simulink model "untitled"  (R2018a)
settings: Solver=ode45  StartTime=0.0  StopTime=1  RelTol=1e-3
libraries: powerlib x4, simulink x2, electricdrivelib x1, spsDrivesSpeedControllerModel x1
settings Model: Creator=HP  LastModifiedBy=HP

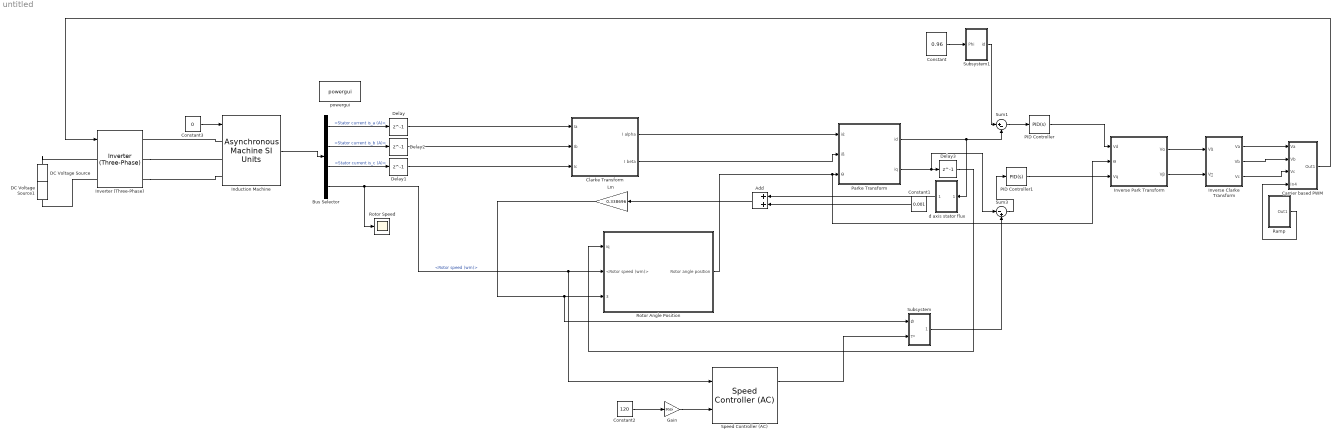
== system untitled ==
  Add : Sum
  Bus Selector : BusSelector  OutputSignals=Stator measurements.Stator current is_a (A),Stator measurements.Stator current is_b (A),Stator measurements.Stator current is_c (A),Mechanical.Rotor speed (wm)
  Carrier based PWM : Subsystem
  Clarke Transform : Subsystem
  Constant : Constant  Value=0.96
  Constant1 : Constant  Value=0.001
  Constant2 : Constant  Value=120
  Constant3 : Constant  Value=0
  DC Voltage Source : powerlib/Electrical Sources/DC Voltage Source  Amplitude=250  Measurements=None
  DC Voltage Source1 : powerlib/Electrical Sources/DC Voltage Source  Amplitude=250  Measurements=None
  Delay{,1..3} (4 alike) : Delay  DelayLength=1  InitialCondition=0
  Gain : Gain  Gain=30/pi
  "Induction Machine " : powerlib/Machines/Asynchronous Machine SI Units  RotorType=Squirrel-cage  PresetModel=No  MechanicalLoad=Torque Tm  ShowDetailedParameters=on  ReferenceFrame=Rotor  Units=SI  MeasurementBus=off  NominalParameters=[1.845e+04 460 50]  Stator=[0.6837 0.004152]  Rotor=[0.451 0.004152]  Cage1=[0.4155 0.002066]  Cage2=[0.4168 0.0003495]  Lm=0.1486  Mechanical=[0.05 0.005879 2]  PolePairs=2  InitialConditions=[1 0 0 0 0 0 0 0]  SimulateSaturation=off  Saturation=[14.03593122, 27.81365428, 53.79336849, 72.68890987, 97.98006896, 148.6815601, 215.7428561, 302.9841135, 428.7778367 ; 230, 322, 414, 460, 506, 552, 598, 644, 690]  LoadFlowParameters=1492000  TsPowergui=0  TsBlock=-1  IterativeModel=Trapezoidal non iterative  IterativeDiscreteModel=Trapezoidal non iterative  Pmec=1.492e+006
  Inverse Clarke Transform : Subsystem
  Inverse Park Transform : Subsystem
  Inverter (Three-Phase) : electricdrivelib/Fundamental Drive Blocks/Inverter (Three-Phase)  OverrideUsingVariant=Detailed  detailLevel=Detailed  driveType=Field-oriented control  Ts=2e-6  SnubberResistance=10e3  SnubberCapacitance=inf  Device=IGBT / Diodes  Ron=1e-3  ForwardVoltages=[1.2,1.2]  GTOparameters=[1e-6,2e-6]  IGBTparameters=[1e-6,2e-6]  Measurements=All voltages and currents  converterType=Inverter  SourceFrequency=60  ReferenceFrame=Rotor  dqInductances=[8.5e-3,8.5e-3]  Inductance=8.5e-3  Ls=0  Resistance=0.2  Flux=0.175  Stator_sm=[2.01e-3,4.289e-4,4.477e-3,1.354e-3]  Stator_im=[14.85e-3,0.3027e-3]  Rotor=[9.295e-3,0.3027e-3]  Lm=10.46e-3  p=4
      settings: AttributesFormatString=%<BlockChoice>  SourceProductName=Simscape Power Systems  SourceProductBaseCode=PS
  Lm : Gain  Gain=0.338696
  PID Controller : simulink/Continuous/PID Controller  Controller=PID  TimeDomain=Continuous-time  SampleTime=-1  IntegratorMethod=Forward Euler  FilterMethod=Forward Euler  Form=Parallel  UseFilter=on  ControllerParametersSource=internal  P=5000  I=200  D=0  N=100  InitialConditionSource=internal  InitialConditionForIntegrator=0  InitialConditionForFilter=0  ExternalReset=none  LimitOutput=off  UpperSaturationLimit=inf  LowerSaturationLimit=-inf  LinearizeAsGain=on  AntiWindupMode=none  Kb=1  TrackingMode=off  Kt=1  PParamMin=[]  PParamMax=[]  IParamMin=[]  IParamMax=[]  DParamMin=[]  DParamMax=[]  NParamMin=[]  NParamMax=[]  KbParamMin=[]  KbParamMax=[]  KtParamMin=[]  KtParamMax=[]  POutMin=[]  POutMax=[]  IOutMin=[]  IOutMax=[]  DOutMin=[]  DOutMax=[]  NOutMin=[]  NOutMax=[]  KbOutMin=[]  KbOutMax=[]  KtOutMin=[]  KtOutMax=[]  IntegratorOutMin=[]  IntegratorOutMax=[]  FilterOutMin=[]  FilterOutMax=[]  SumOutMin=[]  SumOutMax=[]  SumI1OutMin=[]  SumI1OutMax=[]  SumI2OutMin=[]  SumI2OutMax=[]  SumI3OutMin=[]  SumI3OutMax=[]  SumDOutMin=[]  SumDOutMax=[]  SaturationOutMin=[]  SaturationOutMax=[]  IntegratorContinuousStateAttributes=''  IntegratorStateMustResolveToSignalObject=off  IntegratorRTWStateStorageClass=Auto  FilterContinuousStateAttributes=''  FilterStateMustResolveToSignalObject=off  FilterRTWStateStorageClass=Auto  DifferentiatorICPrevScaledInput=0  DifferentiatorOutMin=[]  DifferentiatorOutMax=[]  FilterDiffOutCoefMin=[]  FilterDiffOutCoefMax=[]  SumDenOutMin=[]  SumDenOutMax=[]  SumNumOutMin=[]  SumNumOutMax=[]  ReciprocalOutMin=[]  ReciprocalOutMax=[]  DivideOutMin=[]  DivideOutMax=[]  TunerSelectOption=Transfer Function Based (PID Tuner App)
  PID Controller1 : simulink/Continuous/PID Controller  Controller=PID  TimeDomain=Continuous-time  SampleTime=-1  IntegratorMethod=Forward Euler  FilterMethod=Forward Euler  Form=Parallel  UseFilter=on  ControllerParametersSource=internal  P=5000  I=200  D=0  N=100  InitialConditionSource=internal  InitialConditionForIntegrator=0  InitialConditionForFilter=0  ExternalReset=none  LimitOutput=off  UpperSaturationLimit=inf  LowerSaturationLimit=-inf  LinearizeAsGain=on  AntiWindupMode=none  Kb=1  TrackingMode=off  Kt=1  PParamMin=[]  PParamMax=[]  IParamMin=[]  IParamMax=[]  DParamMin=[]  DParamMax=[]  NParamMin=[]  NParamMax=[]  KbParamMin=[]  KbParamMax=[]  KtParamMin=[]  KtParamMax=[]  POutMin=[]  POutMax=[]  IOutMin=[]  IOutMax=[]  DOutMin=[]  DOutMax=[]  NOutMin=[]  NOutMax=[]  KbOutMin=[]  KbOutMax=[]  KtOutMin=[]  KtOutMax=[]  IntegratorOutMin=[]  IntegratorOutMax=[]  FilterOutMin=[]  FilterOutMax=[]  SumOutMin=[]  SumOutMax=[]  SumI1OutMin=[]  SumI1OutMax=[]  SumI2OutMin=[]  SumI2OutMax=[]  SumI3OutMin=[]  SumI3OutMax=[]  SumDOutMin=[]  SumDOutMax=[]  SaturationOutMin=[]  SaturationOutMax=[]  IntegratorContinuousStateAttributes=''  IntegratorStateMustResolveToSignalObject=off  IntegratorRTWStateStorageClass=Auto  FilterContinuousStateAttributes=''  FilterStateMustResolveToSignalObject=off  FilterRTWStateStorageClass=Auto  DifferentiatorICPrevScaledInput=0  DifferentiatorOutMin=[]  DifferentiatorOutMax=[]  FilterDiffOutCoefMin=[]  FilterDiffOutCoefMax=[]  SumDenOutMin=[]  SumDenOutMax=[]  SumNumOutMin=[]  SumNumOutMax=[]  ReciprocalOutMin=[]  ReciprocalOutMax=[]  DivideOutMin=[]  DivideOutMax=[]  TunerSelectOption=Transfer Function Based (PID Tuner App)
  Parke Transform : Subsystem
  Ramp : Subsystem
  Rotor Angle Position : Subsystem
  "Rotor Speed " : Scope
  Speed Controller (AC) : spsDrivesSpeedControllerModel/Speed Controller (AC)  OverrideUsingVariant=AC345  ctrlType=Without flux reference output  SwK=Speed regulation  Ts=2e-6  ramp=[-18000000000000,18000000000000]  kp=166.2  ki=27700  fc=100  ctrl_sat=[-100,100]  Tsc=100e-6  fn=60  p=2  nf=0.3
      settings: SourceProductName=The database C:\Users\ak23510\AppData\Roaming\MathWorks\MATLAB\R2017a\slblocks_master.db is locked, or a table in the database is locked. (database is locked)
  Subsystem : Subsystem
  Subsystem1 : Subsystem
  Sum1 : Sum  Inputs=|+-
  Sum3 : Sum  Inputs=|-+
  d axis stator flux : Subsystem
  powergui : powerlib/powergui  Priority=1  SimulationMode=Discrete  SampleTime=2e-6  frequency=60  Iterations=50  frequencyindice=50  Pbase=100e6  ErrMax=1e-4  UnitsV=kV  UnitsW=MW  buscounter=0  FunctionMessages=off  echomessages=off  EnableUseOfTLC=off  CurrentSourceSwitches=off  DisableSnubberDevices=off  DisableRonSwitches=off  DisableVfSwitches=off  DisplayEquations=off  SolverType=Tustin/Backward Euler (TBE)  Interpol=off  ExternalGateDelay=off  methode=off  Ts=100  x0status=blocks  SPID=on  SwTol=0  HookPort=off  RestoreLinks=warning  ResistiveCurrentMeasurement=off  Frange=[0:2:500]  Ylog=off  Xlog=on  ShowGrid=off  save=off  variable=ZData  structure=0  ZoomFFT=off  StartTime=0.0  cycles=1  DisplayStyle=1  fundamental=60  FreqAxis=off  MaxFrequency=1000  frequencyindicesteady=1  RmsSteady=1  display=off
  wires:
  "Induction Machine "/1 -> Bus Selector/1
  Bus Selector/1 -> Delay/1  "<Stator current is_a (A)>"
  Bus Selector/2 -> Delay2/1  "<Stator current is_b (A)>"
  Bus Selector/3 -> Delay1/1  "<Stator current is_c (A)>"
  Delay/1 -> Clarke Transform/1(Ia)
  Delay2/1 -> Clarke Transform/2(Ib)
  Delay1/1 -> Clarke Transform/3(Ic)
  Clarke Transform/1(I alpha) -> Parke Transform/1("iά ")
  Clarke Transform/2(I beta) -> Parke Transform/2(iß)
  Parke Transform/1(id) -> d axis stator flux/1(In1), Sum1/2
  d axis stator flux/1(øds) -> Add/1
  Constant1/1 -> Add/2
  Add/1 -> Lm/1
  Bus Selector/4 -> "Rotor Speed "/1, Speed Controller (AC)/1, Rotor Angle Position/2(<Rotor speed (wm)>)  "<Rotor speed (wm)>"
  Lm/1 -> Subsystem/1(Ǿ), Rotor Angle Position/3(" ")
  Rotor Angle Position/1("Rotor angle position ") -> Inverse Park Transform/2(Ɵ), Parke Transform/3(Ɵ)
  Subsystem1/1("id ") -> Sum1/1
  Sum1/1 -> PID Controller/1
  Sum3/1 -> PID Controller1/1
  Subsystem/1(iq ref) -> Sum3/2
  PID Controller/1 -> Inverse Park Transform/1(Vd)
  PID Controller1/1 -> Inverse Park Transform/3(Vq)
  Inverse Park Transform/2(Vβ) -> Inverse Clarke Transform/2(Vꞵ)
  Ramp/1(Out1) -> Carrier based PWM/4(In4)
  Inverse Park Transform/1(Vα) -> Inverse Clarke Transform/1(Vἀ)
  Inverse Clarke Transform/2(Vb) -> Carrier based PWM/2(Vb)
  Inverse Clarke Transform/1(Va) -> Carrier based PWM/1(Va)
  Inverse Clarke Transform/3(Vc) -> Carrier based PWM/3(Vc)
  Carrier based PWM/1(Out1) -> Inverter (Three-Phase)/1
  Constant/1 -> Subsystem1/1(Phi)
  Gain/1 -> Speed Controller (AC)/2
  Constant2/1 -> Gain/1
  Speed Controller (AC)/1 -> Subsystem/2(T*)
  Constant3/1 -> "Induction Machine "/1
  Parke Transform/2(iq) -> Sum3/1, Delay3/1
  Delay3/1 -> Rotor Angle Position/1(iq)
  connections:
  "Induction Machine "/LConn1 -- Inverter (Three-Phase)/RConn1
  Inverter (Three-Phase)/RConn2 -- "Induction Machine "/LConn2
  Inverter (Three-Phase)/RConn3 -- "Induction Machine "/LConn3
  DC Voltage Source1/RConn1 -- DC Voltage Source/LConn1
  DC Voltage Source/RConn1 -- Inverter (Three-Phase)/LConn1
  DC Voltage Source1/LConn1 -- Inverter (Three-Phase)/LConn2

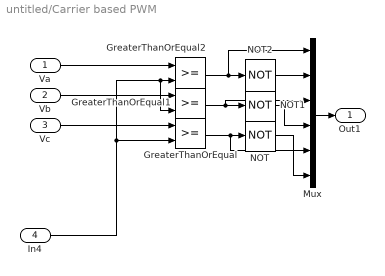
== system untitled/Carrier based PWM ==
  Va : Inport
  Vb : Inport  Port=2
  Vc : Inport  Port=3
  In4 : Inport  Port=4
  GreaterThanOrEqual : RelationalOperator  OutDataTypeStr=boolean  RndMeth=Simplest
  GreaterThanOrEqual1 : RelationalOperator  OutDataTypeStr=boolean  RndMeth=Simplest
  GreaterThanOrEqual2 : RelationalOperator  OutDataTypeStr=boolean  RndMeth=Simplest
  Mux : Mux  Inputs=6
  NOT : Logic  Operator=NOT  IconShape=distinctive  AllPortsSameDT=off  OutDataTypeStr=boolean
  NOT1 : Logic  Operator=NOT  IconShape=distinctive  AllPortsSameDT=off  OutDataTypeStr=boolean
  NOT2 : Logic  Operator=NOT  IconShape=distinctive  AllPortsSameDT=off  OutDataTypeStr=boolean
  Out1 : Outport
  wires:
  GreaterThanOrEqual1/1 -> Mux/3, NOT1/1
  GreaterThanOrEqual2/1 -> Mux/1, NOT2/1
  NOT2/1 -> Mux/2
  NOT1/1 -> Mux/4
  In4/1 -> GreaterThanOrEqual/2, GreaterThanOrEqual1/2, GreaterThanOrEqual2/2
  Va/1 -> GreaterThanOrEqual2/1
  NOT/1 -> Mux/6
  GreaterThanOrEqual/1 -> Mux/5, NOT/1
  Vb/1 -> GreaterThanOrEqual1/1
  Mux/1 -> Out1/1
  Vc/1 -> GreaterThanOrEqual/1

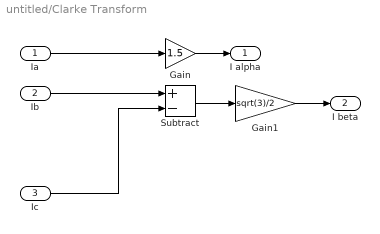
== system untitled/Clarke Transform ==
  Ia : Inport
  Ib : Inport  Port=2
  Ic : Inport  Port=3
  Gain : Gain  Gain=1.5
  Gain1 : Gain  Gain=sqrt(3)/2
  Subtract : Sum  Inputs=+-
  I alpha : Outport
  I beta : Outport  Port=2
  wires:
  Subtract/1 -> Gain1/1
  Ic/1 -> Subtract/2
  Gain1/1 -> I beta/1
  Ia/1 -> Gain/1
  Ib/1 -> Subtract/1
  Gain/1 -> I alpha/1

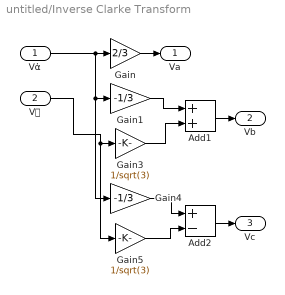
== system untitled/Inverse Clarke Transform ==
  Vἀ : Inport
  Vꞵ : Inport  Port=2
  Add1 : Sum
  Add2 : Sum  Inputs=+-
  Gain : Gain  Gain=2/3
  Gain1 : Gain  Gain=-1/3
  Gain3 : Gain  Gain=1/sqrt(3)
  Gain4 : Gain  Gain=-1/3
  Gain5 : Gain  Gain=1/sqrt(3)
  Va : Outport
  Vb : Outport  Port=2
  Vc : Outport  Port=3
  wires:
  Gain4/1 -> Add2/1
  Vἀ/1 -> Gain1/1, Gain4/1, Gain/1
  Add2/1 -> Vc/1
  Gain1/1 -> Add1/1
  Gain5/1 -> Add2/2
  Gain3/1 -> Add1/2
  Vꞵ/1 -> Gain5/1, Gain3/1
  Add1/1 -> Vb/1
  Gain/1 -> Va/1

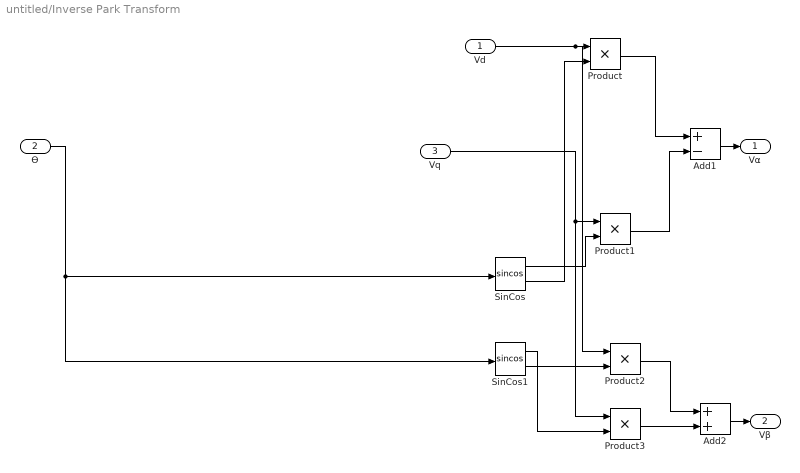
== system untitled/Inverse Park Transform ==
  Vd : Inport
  Ɵ : Inport  Port=2
  Vq : Inport  Port=3
  Add1 : Sum  Inputs=+-
  Add2 : Sum
  Product{,1..3} (4 alike) : Product
  SinCos : Trigonometry  Operator=sincos
  SinCos1 : Trigonometry  Operator=sincos
  Vα : Outport
  Vβ : Outport  Port=2
  wires:
  Product2/1 -> Add2/1
  SinCos1/2 -> Product2/2
  Ɵ/1 -> SinCos1/1, SinCos/1
  Vd/1 -> Product2/1, Product/1
  SinCos/1 -> Product1/2
  SinCos/2 -> Product/2
  Vq/1 -> Product3/1, Product1/1
  Product3/1 -> Add2/2
  Product/1 -> Add1/1
  SinCos1/1 -> Product3/2
  Product1/1 -> Add1/2
  Add1/1 -> Vα/1
  Add2/1 -> Vβ/1

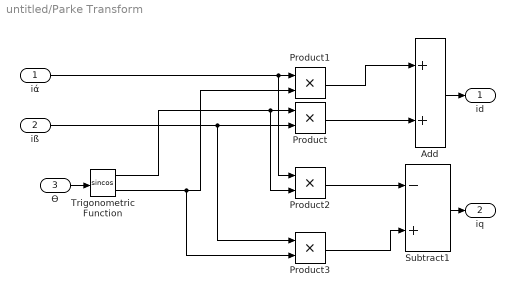
== system untitled/Parke Transform ==
  "iά " : Inport
  iß : Inport  Port=2
  Ɵ : Inport  Port=3
  Add : Sum
  Product{,1..3} (4 alike) : Product
  Subtract1 : Sum  Inputs=-+
  Trigonometric Function : Trigonometry  Operator=sincos
  id : Outport
  iq : Outport  Port=2
  wires:
  Trigonometric Function/1 -> Product2/2, Product/1
  "iά "/1 -> Product2/1, Product1/1
  iß/1 -> Product3/1, Product/2
  Trigonometric Function/2 -> Product1/2, Product3/2
  Product/1 -> Add/2
  Product1/1 -> Add/1
  Add/1 -> id/1
  Ɵ/1 -> Trigonometric Function/1
  Subtract1/1 -> iq/1
  Product2/1 -> Subtract1/1
  Product3/1 -> Subtract1/2

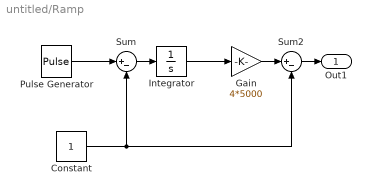
== system untitled/Ramp ==
  Constant : Constant
  Gain : Gain  Gain=4*5000
  Integrator : Integrator
  Pulse Generator : DiscretePulseGenerator  PulseType=Time based  Amplitude=2  Period=1/5000  PulseWidth=50
  Sum : Sum  Inputs=|+-
  Sum2 : Sum  Inputs=|+-
  Out1 : Outport
  wires:
  Gain/1 -> Sum2/1
  Integrator/1 -> Gain/1
  Sum2/1 -> Out1/1
  Pulse Generator/1 -> Sum/1
  Constant/1 -> Sum2/2, Sum/2
  Sum/1 -> Integrator/1

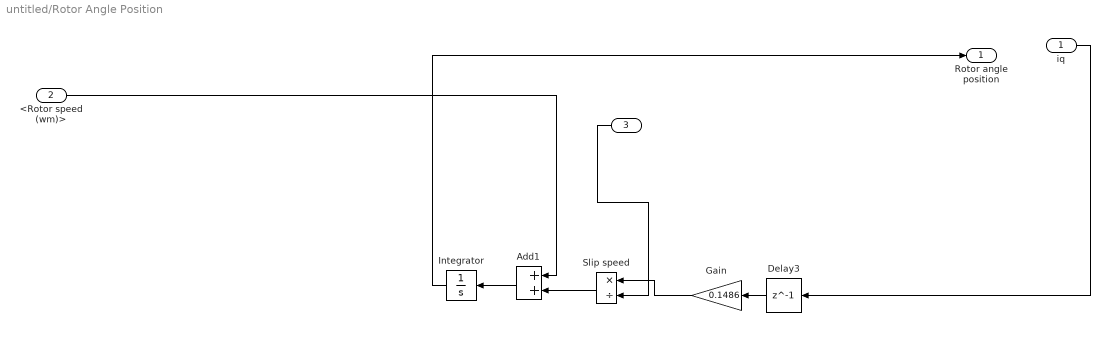
== system untitled/Rotor Angle Position ==
  iq : Inport
  <Rotor speed (wm)> : Inport  Port=2
  " " : Inport  Port=3
  Add1 : Sum
  Delay3 : Delay  DelayLength=1  InitialCondition=0
  Gain : Gain  Gain=0.1486
  Integrator : Integrator
  Slip speed : Product  Inputs=*/
  "Rotor angle position " : Outport
  wires:
  Gain/1 -> Slip speed/1
  Add1/1 -> Integrator/1
  Integrator/1 -> "Rotor angle position "/1
  Slip speed/1 -> Add1/2
  Delay3/1 -> Gain/1
  iq/1 -> Delay3/1
  " "/1 -> Slip speed/2
  <Rotor speed (wm)>/1 -> Add1/1

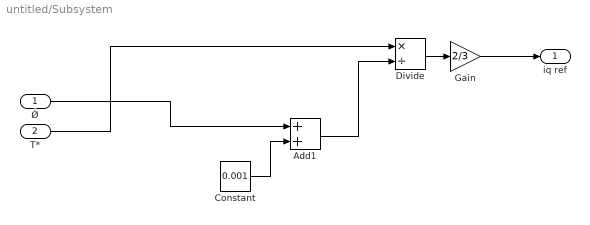
== system untitled/Subsystem ==
  Ǿ : Inport
  T* : Inport  Port=2
  Add1 : Sum
  Constant : Constant  Value=0.001
  Divide : Product  Inputs=*/
  Gain : Gain  Gain=2/3
  iq ref : Outport
  wires:
  Add1/1 -> Divide/2
  Gain/1 -> iq ref/1
  Divide/1 -> Gain/1
  Constant/1 -> Add1/2
  T*/1 -> Divide/1
  Ǿ/1 -> Add1/1

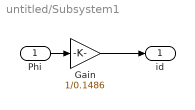
== system untitled/Subsystem1 ==
  Phi : Inport
  Gain : Gain  Gain=1/0.1486
  "id " : Outport
  wires:
  Phi/1 -> Gain/1
  Gain/1 -> "id "/1

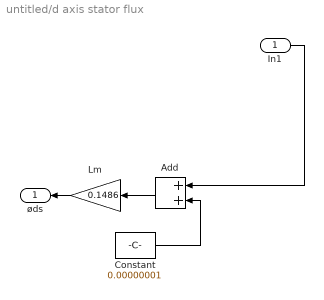
== system untitled/d axis stator flux ==
  In1 : Inport
  Add : Sum
  Constant : Constant  Value=0.00000001
  Lm : Gain  Gain=0.1486
  øds : Outport
  wires:
  In1/1 -> Add/1
  Add/1 -> Lm/1
  Lm/1 -> øds/1
  Constant/1 -> Add/2
